simulink model "estados_test"  (R2020b)
settings: Solver=VariableStepAuto  StartTime=0.0  StopTime=100  RelTol=1e-3
settings Model: Creator=jlanzas  LastModifiedBy=Juan

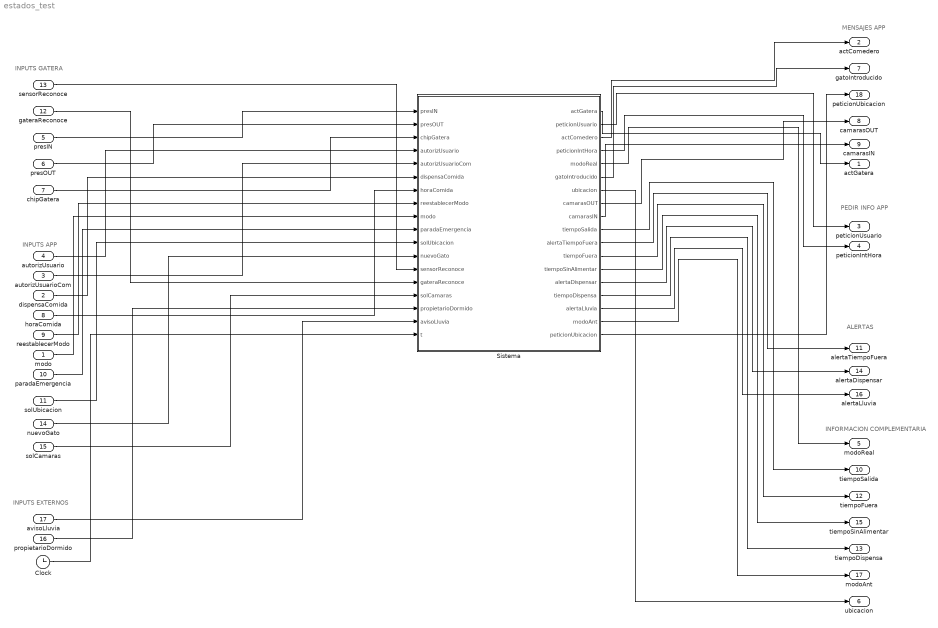
== system estados_test ==
  note: INFORMACION COMPLEMENTARIA
  note: ALERTAS
  note: PEDIR INFO APP
  note: INPUTS EXTERNOS
  note: INPUTS APP
  note: MENSAJES APP
  note: INPUTS GATERA
  modo : Inport
  dispensaComida : Inport  Port=2
  autorizUsuarioCom : Inport  Port=3
  autorizUsuario : Inport  Port=4
  presIN : Inport  Port=5
  presOUT : Inport  Port=6
  chipGatera : Inport  Port=7
  horaComida : Inport  Port=8
  reestablecerModo : Inport  Port=9
  paradaEmergencia : Inport  Port=10
  solUbicacion : Inport  Port=11
  gateraReconoce : Inport  Port=12
  sensorReconoce : Inport  Port=13
  nuevoGato : Inport  Port=14
  solCamaras : Inport  Port=15
  propietarioDormido : Inport  Port=16
  avisoLluvia : Inport  Port=17
  Clock : Clock
  Sistema : Stateflow chart  TreatAsAtomicUnit=on
  actGatera : Outport
  actComedero : Outport  Port=2
  peticionUsuario : Outport  Port=3
  peticionIntHora : Outport  Port=4
  modoReal : Outport  Port=5
  ubicacion : Outport  Port=6
  gatoIntroducido : Outport  Port=7
  camarasOUT : Outport  Port=8
  camarasIN : Outport  Port=9
  tiempoSalida : Outport  Port=10
  alertaTiempoFuera : Outport  Port=11
  tiempoFuera : Outport  Port=12
  tiempoDispensa : Outport  Port=13
  alertaDispensar : Outport  Port=14
  tiempoSinAlimentar : Outport  Port=15
  alertaLluvia : Outport  Port=16
  modoAnt : Outport  Port=17
  peticionUbicacion : Outport  Port=18
  wires:
  Sistema/1(actGatera) -> actGatera/1
  autorizUsuario/1 -> Sistema/4(autorizUsuario)
  autorizUsuarioCom/1 -> Sistema/5(autorizUsuarioCom)
  dispensaComida/1 -> Sistema/6(dispensaComida)
  presIN/1 -> Sistema/1(presIN)
  presOUT/1 -> Sistema/2(presOUT)
  chipGatera/1 -> Sistema/3(chipGatera)
  Sistema/2(peticionUsuario) -> peticionUsuario/1
  horaComida/1 -> Sistema/7(horaComida)
  Sistema/4(peticionIntHora) -> peticionIntHora/1
  reestablecerModo/1 -> Sistema/8(reestablecerModo)
  modo/1 -> Sistema/9(modo)
  Sistema/3(actComedero) -> actComedero/1
  Sistema/5(modoReal) -> modoReal/1
  paradaEmergencia/1 -> Sistema/10(paradaEmergencia)
  Sistema/7(ubicacion) -> ubicacion/1
  solUbicacion/1 -> Sistema/11(solUbicacion)
  gateraReconoce/1 -> Sistema/14(gateraReconoce)
  sensorReconoce/1 -> Sistema/13(sensorReconoce)
  nuevoGato/1 -> Sistema/12(nuevoGato)
  Sistema/6(gatoIntroducido) -> gatoIntroducido/1
  solCamaras/1 -> Sistema/15(solCamaras)
  Sistema/8(camarasOUT) -> camarasOUT/1
  Sistema/9(camarasIN) -> camarasIN/1
  Sistema/10(tiempoSalida) -> tiempoSalida/1
  Sistema/11(alertaTiempoFuera) -> alertaTiempoFuera/1
  Sistema/12(tiempoFuera) -> tiempoFuera/1
  Sistema/14(alertaDispensar) -> alertaDispensar/1
  Sistema/15(tiempoDispensa) -> tiempoDispensa/1
  Sistema/13(tiempoSinAlimentar) -> tiempoSinAlimentar/1
  propietarioDormido/1 -> Sistema/16(propietarioDormido)
  Sistema/16(alertaLluvia) -> alertaLluvia/1
  avisoLluvia/1 -> Sistema/17(avisoLluvia)
  Sistema/17(modoAnt) -> modoAnt/1
  Clock/1 -> Sistema/18(t)
  Sistema/18(peticionUbicacion) -> peticionUbicacion/1

== stateflow chart estados_test/Sistema ==
  state App [parallel]
    settings: executionOrder=3
    state ModoUso
      state Bloqueo
        entry:
        modoReal=2;
      state Auto
        entry:
        peticionIntHora=0;
        modoReal=0;
      state Manual
        entry:
        modoReal=1;
      App.ModoUso.Manual -> App.ModoUso.Bloqueo [order 1] : [paradaEmergencia==1]{modoAnt=1;}
      App.ModoUso.Auto -> App.ModoUso.Bloqueo [order 1] : [paradaEmergencia==1]{modoAnt=0;}
      App.ModoUso.Bloqueo -> (junction 379) : [reestablecerModo==1]
      (junction 379) -> App.ModoUso.Manual [order 1] : [modoAnt==1]
      (junction 379) -> App.ModoUso.Auto [order 2] : [modoAnt==0]
      (default) -> App.ModoUso.Manual
      App.ModoUso.Auto -> App.ModoUso.Manual [order 2] : [modo==1]
      (junction 368) -> App.ModoUso.Auto [order 1] : [horaComida~=0]
      (junction 368) -> App.ModoUso.Manual [order 2] : [horaComida==0]
      App.ModoUso.Manual -> (junction 365) [order 2] : [modo==0]
      (junction 365) -> (junction 368) : {peticionIntHora=1;}
    state SolicitudUbicacion
      entry:
      peticionUbicacion=ubicacion;
    state InsertarGato
      state ReconocimientoGatera
      state ReconocimientoSensor
      state GatoNuevo
        gatoIntroducido=1;
      (default) -> ReconocimientoGatera
      ReconocimientoGatera -> ReconocimientoSensor : [gateraReconoce==1]
      ReconocimientoSensor -> GatoNuevo : [sensorReconoce==1]
    (default) -> ModoUso
    ModoUso -> SolicitudUbicacion [order 1] : [solUbicacion==1]
    ModoUso -> InsertarGato [order 2] : [nuevoGato==1]
    SolicitudUbicacion -> SolicitudUbicacion [order 2] : [solUbicacion==1]
    SolicitudUbicacion -> (junction 459) [order 1] : [solCamaras==1]
  state EstadisticasComida [parallel]
    settings: executionOrder=6
    state Inicio
      entry: tiempoDispensa=0;
      alertaDispensar=0;
    state ExcesoSinDispensar
      entry: alertaDispensar=1;
      tiempoSinAlimentar=t-tiempoDispensa;
    state GatoAlimentado1
      entry: tiempoSinAlimentar=t-tiempoDispensa;
      alertaDispensar=0;
    (default) -> Inicio
    Inicio -> GatoAlimentado1 : [tiempoDispensa~=0]
    GatoAlimentado1 -> ExcesoSinDispensar [order 2] : [tiempoSinAlimentar>=25]
    GatoAlimentado1 -> GatoAlimentado1 [order 1] : [tiempoSinAlimentar<25]
    ExcesoSinDispensar -> GatoAlimentado1 [order 1] : [tiempoSinAlimentar<25]
    ExcesoSinDispensar -> ExcesoSinDispensar [order 2] : [tiempoSinAlimentar>=25]
  state EstadisticasUbicacion [parallel]
    settings: executionOrder=5
    state GatoDentro
      entry: tiempoSalida=0;
    state TiempoFuera
      entry: tiempoFuera=t-tiempoSalida;
    state ExcesoTiempoFuera
      entry: alertaTiempoFuera=1;
    (default) -> GatoDentro
    TiempoFuera -> GatoDentro [order 3] : [tiempoSalida==0]
    GatoDentro -> TiempoFuera : [tiempoSalida~=0]
    TiempoFuera -> ExcesoTiempoFuera [order 2] : [tiempoFuera>=20]
    TiempoFuera -> TiempoFuera [order 1] : [tiempoFuera<20]
  state AlertaDeLluvia [parallel]
    settings: executionOrder=7
    state SinAvisoDeLluvia
      alertaLluvia=0;
    state AvisoDeLluvia
      alertaLluvia=1;
    (default) -> SinAvisoDeLluvia
    SinAvisoDeLluvia -> AvisoDeLluvia : [avisoLluvia==1]
    AvisoDeLluvia -> SinAvisoDeLluvia : [avisoLluvia==0]
  state Camaras [parallel]
    settings: executionOrder=4
    state solCamarasIN
      entry:
      camarasIN=1;
    state solCamarasOUT
      entry:
      camarasOUT=1;
    state CamarasOFF
    (default) -> CamarasOFF
  state Gatera [parallel]
    settings: executionOrder=1
    state Manual
      state AbiertoFuera
        entry: actGatera=1;
      state Cerrado
        entry: actGatera=0;
        peticionUsuario=0;
      state CerradoNoDetectarF
        entry: actGatera=0;
      state GatoCruzando1
      state HaEntrado
        entry: ubicacion=1;
      state GatoHaCruzado1
        entry: tiempoSalida=0.0;
        alertaTiempoFuera=0;
      state HaSalido
        entry:ubicacion=0;
      state Espera
        entry: peticionUsuario=1
      state CerradoNoDetectarD
        entry: actGatera=0;
      state GatoHaCruzado
        entry: tiempoSalida=t;
      state GatoCruzando
      state AbiertoDentro1
        entry: actGatera=1;
        peticionUsuario=0;
      Gatera.Manual.AbiertoFuera -> Gatera.Manual.Cerrado [order 2] : [presOUT==0]
      (default) -> Gatera.Manual.Cerrado
      Gatera.Manual.AbiertoFuera -> Gatera.Manual.GatoCruzando1 [order 1] : [chipGatera==1]
      Gatera.Manual.Cerrado -> Gatera.Manual.AbiertoFuera [order 1] : [presOUT==1]
      Gatera.Manual.AbiertoFuera -> Gatera.Manual.CerradoNoDetectarF [order 3] : after(10,sec)
      Gatera.Manual.GatoCruzando1 -> Gatera.Manual.AbiertoFuera [order 2] : [chipGatera==1&&presOUT==1]
      Gatera.Manual.CerradoNoDetectarD -> Gatera.Manual.Cerrado : after(30,sec)
      Gatera.Manual.HaSalido -> Gatera.Manual.Cerrado
      AbiertoDentro1 -> Gatera.Manual.Cerrado [order 3] : [presIN==0]
      Gatera.Manual.Cerrado -> Espera [order 2] : [presIN==1]
      Espera -> Gatera.Manual.Cerrado [order 1] : [presIN==0]
      Gatera.Manual.HaEntrado -> Gatera.Manual.Cerrado
      Gatera.Manual.CerradoNoDetectarF -> Gatera.Manual.Cerrado : after(30,sec)
      Gatera.Manual.GatoCruzando1 -> Gatera.Manual.GatoHaCruzado1 [order 1] : [chipGatera==0&&presOUT==0]
      Gatera.Manual.GatoHaCruzado1 -> Gatera.Manual.GatoCruzando1 [order 1] : [chipGatera==1]
      Gatera.Manual.GatoHaCruzado1 -> Gatera.Manual.HaEntrado [order 2] : after(10,sec)
      Gatera.Manual.GatoHaCruzado -> Gatera.Manual.HaSalido [order 2] : after(10,sec)
      Espera -> AbiertoDentro1 [order 2] : [autorizUsuario==1]
      Gatera.Manual.GatoHaCruzado -> Gatera.Manual.GatoCruzando [order 1] : [chipGatera==1]
      Gatera.Manual.GatoCruzando -> Gatera.Manual.GatoHaCruzado [order 1] : [chipGatera==0&presIN==0]
      AbiertoDentro1 -> Gatera.Manual.CerradoNoDetectarD [order 1] : after(10,sec)
      Gatera.Manual.GatoCruzando -> AbiertoDentro1 [order 2] : [chipGatera==0&presIN==1]
      AbiertoDentro1 -> Gatera.Manual.GatoCruzando [order 2] : [chipGatera==1]
    state Inicializador
      ubicacion=1;
    state Auto
      state Cerrado
        entry: actGatera=0;
      state AbiertoFuera
        entry: actGatera=1;
      state CerradoNoDetectarF
        entry: actGatera=0;
      state GatoCruzando1
      state HaEntrado
        entry: ubicacion=1;
      state GatoHaCruzado1
        tiempoSalida = 0.0;
        alertaTiempoFuera=0;
      state HaSalido
        entry: ubicacion=0;
      state CerradoNoDetectarD
        entry: actGatera=0;
      state GatoHaCruzado
        tiempoSalida = t;
      state GatoCruzando
      state AbiertoDentro
        entry: actGatera=1;
      Gatera.Auto.Cerrado -> Gatera.Auto.AbiertoFuera [order 1] : [presOUT==1]
      (default) -> Gatera.Auto.Cerrado
      Gatera.Auto.AbiertoFuera -> Gatera.Auto.Cerrado [order 2] : [presOUT==0]
      Gatera.Auto.CerradoNoDetectarF -> Gatera.Auto.Cerrado : after(30,sec)
      Gatera.Auto.AbiertoFuera -> Gatera.Auto.CerradoNoDetectarF [order 3] : after(10,sec)
      Gatera.Auto.CerradoNoDetectarD -> Gatera.Auto.Cerrado : after(30,sec)
      Gatera.Auto.HaSalido -> Gatera.Auto.Cerrado
      AbiertoDentro -> Gatera.Auto.Cerrado [order 2] : [presIN==0]
      Gatera.Auto.Cerrado -> AbiertoDentro [order 2] : [presIN==1]
      Gatera.Auto.HaEntrado -> Gatera.Auto.Cerrado
      Gatera.Auto.GatoCruzando1 -> Gatera.Auto.AbiertoFuera [order 2] : [chipGatera==0&presOUT==1]
      Gatera.Auto.AbiertoFuera -> Gatera.Auto.GatoCruzando1 [order 1] : [chipGatera==1]
      Gatera.Auto.GatoHaCruzado1 -> Gatera.Auto.GatoCruzando1 [order 1] : [chipGatera==1]
      Gatera.Auto.GatoCruzando1 -> Gatera.Auto.GatoHaCruzado1 [order 1] : [chipGatera==0&presOUT==0]
      Gatera.Auto.GatoHaCruzado1 -> Gatera.Auto.HaEntrado [order 2] : after(10,sec)
      AbiertoDentro -> Gatera.Auto.CerradoNoDetectarD [order 3] : after(10,sec)
      Gatera.Auto.GatoHaCruzado -> Gatera.Auto.HaSalido [order 2] : after(10,sec)
      Gatera.Auto.GatoHaCruzado -> Gatera.Auto.GatoCruzando [order 1] : [chipGatera==1]
      Gatera.Auto.GatoCruzando -> Gatera.Auto.GatoHaCruzado [order 1] : [chipGatera==0&presIN==0]
      Gatera.Auto.GatoCruzando -> AbiertoDentro [order 2] : [chipGatera==0&presIN==1]
      AbiertoDentro -> Gatera.Auto.GatoCruzando [order 1] : [chipGatera==1]
    state Bloqueo
      entry: actGatera=0
    (default) -> Inicializador
    Inicializador -> Gatera.Auto
    Gatera.Auto -> Gatera.Manual [order 1] : [modoReal==1]
    Gatera.Manual -> Gatera.Auto [order 2] : [modoReal==0]
    Gatera.Bloqueo -> Gatera.Auto [order 1] : [modoReal==0]
    Gatera.Auto -> Gatera.Bloqueo [order 2] : [modoReal==2]
    Gatera.Manual -> Gatera.Bloqueo [order 1] : [modoReal==2]
    Gatera.Bloqueo -> Gatera.Manual [order 2] : [modoReal==1]
  state Comedero [parallel]
    settings: executionOrder=2
    state Manual
      state Inactivo
        entry: actComedero=0;
      state Dispensa
        entry: actComedero=1
        tiempoDispensa=t;
        %alertaDispensar=0;
      (default) -> Comedero.Manual.Inactivo
      Comedero.Manual.Inactivo -> Comedero.Manual.Dispensa [order 1] : [propietarioDormido==1]
      Comedero.Manual.Inactivo -> Comedero.Manual.Dispensa [order 2] : [autorizUsuarioCom==1]
      Comedero.Manual.Dispensa -> Comedero.Manual.Inactivo : after(10,'sec')
    state Auto
      state Inactivo
        entry: actComedero=0;
      state Dispensa
        entry: actComedero=1
      (default) -> Comedero.Auto.Inactivo
      Comedero.Auto.Inactivo -> Comedero.Auto.Dispensa : [t>=horaComida&&t<(horaComida+10)]
      Comedero.Auto.Dispensa -> Comedero.Auto.Inactivo : after(10,'sec')
    (default) -> Comedero.Auto
    Comedero.Manual -> Comedero.Auto : [modoReal==0]
    Comedero.Auto -> Comedero.Manual : [modoReal~=0]
  (junction 459) -> solCamarasOUT [order 2] : [ubicacion==0]
  (junction 459) -> solCamarasIN [order 1] : [ubicacion==1]
  data: presIN input; presOUT input; actGatera output; chipGatera input; autorizUsuario input; peticionUsuario output; actComedero output; autorizUsuarioCom input; dispensaComida input; horaComida input; peticionIntHora output; reestablecerModo input; modo input; modoReal output; paradaEmergencia input; solUbicacion input; nuevoGato input; sensorReconoce input; gateraReconoce input; gatoIntroducido output; ubicacion output; camarasOUT output; camarasIN output; solCamaras input; tiempoSalida output; alertaTiempoFuera output; tiempoFuera output; tiempoSinAlimentar output; alertaDispensar output; tiempoDispensa output; propietarioDormido input; avisoLluvia input; alertaLluvia output; modoAnt output; t input; peticionUbicacion output
